simulink model "cps_physics_v2"  (R2012b)
settings: Solver=FixedStepDiscrete  StartTime=0.0  StopTime=8.5  FixedStep=0.005  RelTol=1e-5
model workspace (MAT data in the model file):
  nozzle_radius = 0.06
  block_mass = 0.0075
  block_width = 0.15
  ini_G_block_hpos = -0.4
  ini_G_block_vpos = 0.11
  ini_nozzle_pos = 0.3
  block_height = 0.1
  board_vpos = -0.1
  ini_R_block_hpos = -0.4
  ini_R_block_vpos = 0.01
  ini_B_block_vpos = 0.21
  ini_B_block_hpos = -0.4
libraries: fl_lib x52, nesl_utility x19, cps_physics_lib x4, cps_lib_v2 x3
settings Model: Creator=pmosterm  LastModifiedBy=pmosterm
settings SolverCC: MaxConsecutiveZCs=100  EnableConcurrentExecution=on  ConcurrentTasks=on  ZeroCrossAlgorithm=Adaptive
settings DataIOCC: SignalLoggingSaveFormat=ModelDataLogs  SaveOutput=off  DSMLogging=off  SaveTime=off
settings OptimizationCC: InlineParams=on
settings DebuggingCC: ReadBeforeWriteMsg=DisableAll  WriteAfterWriteMsg=DisableAll  WriteAfterReadMsg=DisableAll  AlgebraicLoopMsg=error  UnderspecifiedInitializationDetection=Simplified  FcnCallInpInsideContextMsg=EnableAllAsWarning  ModelReferenceExtraNoncontSigs=warning
settings GRTTargetCC: CombineOutputUpdateFcns=off  GRTInterface=on

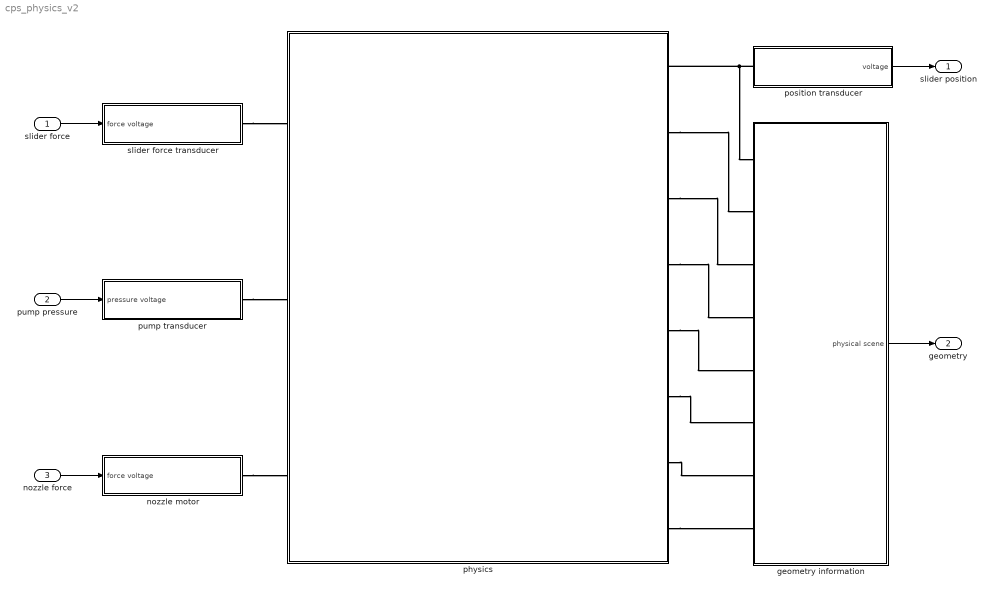
== system cps_physics_v2 ==
  slider force : Inport  SampleTime=[0 1]
  pump pressure : Inport  Port=2
  nozzle force : Inport  Port=3
  geometry information : Subsystem
  nozzle motor : Subsystem
  physics : Subsystem
      settings: OpenFcn=open_system(gcb,'force');
      mask Display: image(imread('images\geo_ton_428x599.jpg'));
  position transducer : Subsystem
  pump transducer : Subsystem
  slider force transducer : Subsystem
  slider position : Outport
  geometry : Outport  Port=2  OutDataTypeStr=Bus: slBusGeometry  BusOutputAsStruct=on
  wires:
  slider force/1 -> slider force transducer/1(force voltage)
  nozzle force/1 -> nozzle motor/1(force voltage)
  pump pressure/1 -> pump transducer/1(pressure voltage)
  geometry information/1(physical scene) -> geometry/1
  position transducer/1(voltage) -> slider position/1
  connections:
  position transducer/LConn1 -- physics/RConn1 -- geometry information/LConn1
  nozzle motor/RConn1 -- physics/LConn3
  physics/RConn4 -- geometry information/LConn4
  physics/RConn3 -- geometry information/LConn3
  slider force transducer/RConn1 -- physics/LConn1
  pump transducer/RConn1 -- physics/LConn2
  physics/RConn2 -- geometry information/LConn2
  physics/RConn5 -- geometry information/LConn5
  physics/RConn6 -- geometry information/LConn6
  physics/RConn7 -- geometry information/LConn7
  physics/RConn8 -- geometry information/LConn8

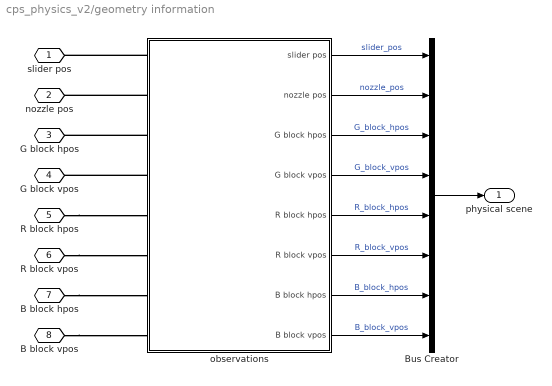
== system cps_physics_v2/geometry information ==
  Bus Creator : BusCreator  Inputs='slider_pos','nozzle_pos','G_block_hpos','G_block_vpos','R_block_hpos','R_block_vpos','B_block_hpos','B_block_vpos'
  observations : Subsystem
  slider pos : PMIOPort  Port=1  Side=Left
  nozzle pos : PMIOPort  Port=2  Side=Left
  G block hpos : PMIOPort  Port=3  Side=Left
  G block vpos : PMIOPort  Port=4  Side=Left
  R block hpos : PMIOPort  Port=5  Side=Left
  R block vpos : PMIOPort  Port=6  Side=Left
  B block hpos : PMIOPort  Port=7  Side=Left
  B block vpos : PMIOPort  Port=8  Side=Left
  physical scene : Outport  OutDataTypeStr=Bus: slBusGeometry
  wires:
  Bus Creator/1 -> physical scene/1
  observations/2(nozzle pos) -> Bus Creator/2  "nozzle_pos"
  observations/3(G block hpos) -> Bus Creator/3  "G_block_hpos"
  observations/4(G block vpos) -> Bus Creator/4  "G_block_vpos"
  observations/1(slider pos) -> Bus Creator/1  "slider_pos"
  observations/5(R block hpos) -> Bus Creator/5  "R_block_hpos"
  observations/6(R block vpos) -> Bus Creator/6  "R_block_vpos"
  observations/7(B block hpos) -> Bus Creator/7  "B_block_hpos"
  observations/8(B block vpos) -> Bus Creator/8  "B_block_vpos"
  connections:
  observations/LConn4 -- G block vpos/RConn1
  observations/LConn3 -- G block hpos/RConn1
  observations/LConn1 -- slider pos/RConn1
  observations/LConn2 -- nozzle pos/RConn1
  R block vpos/RConn1 -- observations/LConn6
  R block hpos/RConn1 -- observations/LConn5
  B block hpos/RConn1 -- observations/LConn7
  B block vpos/RConn1 -- observations/LConn8

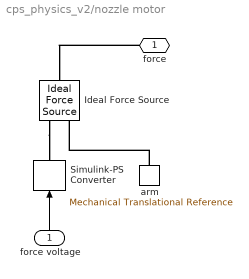
== system cps_physics_v2/nozzle motor ==
  force voltage : Inport
  Ideal Force Source : fl_lib/Mechanical/Mechanical Sources/Ideal Force Source  v_Log=off  f_Log=off  LocalVarNames=|v|f  LocalVarDescs=|v|f  LocalVarLogging=[0 0]
  Simulink-PS Converter : nesl_utility/Simulink-PS Converter  PhysicalDomain=network_engine_domain  LeftPortType=input  RightPortType=output  SubClassName=ps_input  PseudoPeriodic=off  Frequencies=[]  NoiseDistribution=none  NoiseParameters=[]  Unit=1  AffineConversion=off  InputFilterTimeConstant=.001  UdotUserProvided=0  SimscapeFilterOrder=1  InputFiltering=off
  arm : fl_lib/Mechanical/Translational Elements/Mechanical Translational Reference  f_Log=off  LocalVarNames=|f  LocalVarDescs=|f  LocalVarLogging=0
  force : PMIOPort  Port=1  Side=Right
  wires:
  force voltage/1 -> Simulink-PS Converter/1
  connections:
  Ideal Force Source/RConn1 -- Simulink-PS Converter/RConn1
  force/RConn1 -- Ideal Force Source/LConn1
  arm/LConn1 -- Ideal Force Source/RConn2

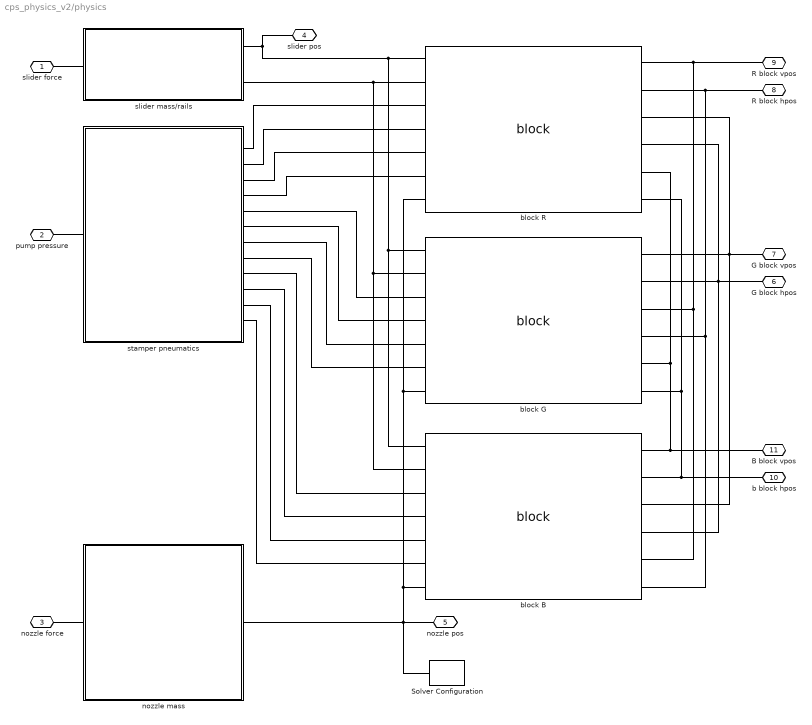
== system cps_physics_v2/physics ==
  Solver Configuration : nesl_utility/Solver Configuration  PhysicalDomain=network_engine_domain  LeftPortType=input  RightPortType=generic  SubClassName=solver  Accelerate=off  Profile=off  UseLocalSampling=off  FrequencyDomain=off  Tones=[]  Harmonics=[]  UseCCode=off  SimulateNoise=off  EnableSwitchedLinearOptims=on  DoDC=off  ResidualTolerance=1e-9  UseLocalSolver=on  LocalSolverChoice=NE_BACKWARD_EULER_ADVANCER  LocalSolverSampleTime=.005  DoFixedCost=on  MaxNonlinIter=3  MaxModeIter=2  LinearAlgebra=Sparse  DelaysMemoryBudget=1024
  block B : cps_lib_v2/block  ini_block_vpos=ini_B_block_vpos  ini_block_hpos=ini_B_block_hpos
  block G : cps_lib_v2/block  ini_block_vpos=ini_G_block_vpos  ini_block_hpos=ini_G_block_hpos
  block R : cps_lib_v2/block  ini_block_vpos=ini_R_block_vpos  ini_block_hpos=ini_R_block_hpos
  nozzle mass : Subsystem
      settings: OpenFcn=open_system(gcb,'force');
      mask Display: image(imread('images\geo_ton_slider_nozzle_202x195.jpg'));
  slider mass/rails : Subsystem
      settings: OpenFcn=open_system(gcb,'force');
      mask Display: image(imread('images\geo_ton_slider_rails_202x88.jpg'));
  stamper pneumatics : Subsystem
      settings: OpenFcn=open_system(gcb,'force');
      mask Display: image(imread('images\geo_ton_pneumatics_202x264.jpg'));
  slider force : PMIOPort  Port=1  Side=Left
  pump pressure : PMIOPort  Port=2  Side=Left
  nozzle force : PMIOPort  Port=3  Side=Left
  slider pos : PMIOPort  Port=4  Side=Right
  nozzle pos : PMIOPort  Port=5  Side=Right
  G block hpos : PMIOPort  Port=6  Side=Right
  G block vpos : PMIOPort  Port=7  Side=Right
  R block hpos : PMIOPort  Port=8  Side=Right
  R block vpos : PMIOPort  Port=9  Side=Right
  b block hpos : PMIOPort  Port=10  Side=Right
  B block vpos : PMIOPort  Port=11  Side=Right
  connections:
  slider mass/rails/RConn1 -- block R/LConn1 -- block B/LConn1 -- block G/LConn1 -- slider pos/RConn1
  slider force/RConn1 -- slider mass/rails/LConn1
  pump pressure/RConn1 -- stamper pneumatics/LConn1
  nozzle force/RConn1 -- nozzle mass/LConn1
  G block hpos/RConn1 -- block B/RConn4 -- block G/RConn2 -- block R/RConn4
  block R/LConn2 -- slider mass/rails/RConn2 -- block B/LConn2 -- block G/LConn2
  R block vpos/RConn1 -- block R/RConn1 -- block B/RConn5 -- block G/RConn3
  R block hpos/RConn1 -- block R/RConn2 -- block B/RConn6 -- block G/RConn4
  G block vpos/RConn1 -- block B/RConn3 -- block G/RConn1 -- block R/RConn3
  nozzle pos/RConn1 -- Solver Configuration/RConn1 -- nozzle mass/RConn1 -- block G/LConn7 -- block R/LConn7 -- block B/LConn7
  block G/LConn3 -- stamper pneumatics/RConn5
  block G/LConn4 -- stamper pneumatics/RConn6
  block G/LConn5 -- stamper pneumatics/RConn7
  block G/LConn6 -- stamper pneumatics/RConn8
  block R/LConn5 -- stamper pneumatics/RConn3
  block R/LConn3 -- stamper pneumatics/RConn1
  block R/LConn4 -- stamper pneumatics/RConn2
  block R/LConn6 -- stamper pneumatics/RConn4
  block B/LConn3 -- stamper pneumatics/RConn9
  block B/LConn4 -- stamper pneumatics/RConn10
  block B/LConn5 -- stamper pneumatics/RConn11
  block B/LConn6 -- stamper pneumatics/RConn12
  B block vpos/RConn1 -- block G/RConn5 -- block R/RConn5 -- block B/RConn1
  b block hpos/RConn1 -- block G/RConn6 -- block R/RConn6 -- block B/RConn2

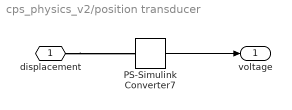
== system cps_physics_v2/position transducer ==
  PS-Simulink Converter7 : nesl_utility/PS-Simulink Converter  PhysicalDomain=network_engine_domain  LeftPortType=input  RightPortType=output  SubClassName=ps_output  PseudoPeriodic=off  Frequencies=[]  Unit=1  AffineConversion=off
  displacement : PMIOPort  Port=1  Side=Left
  voltage : Outport
  wires:
  PS-Simulink Converter7/1 -> voltage/1
  connections:
  displacement/RConn1 -- PS-Simulink Converter7/LConn1

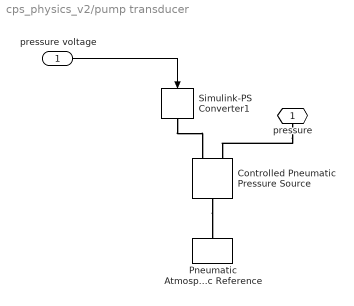
== system cps_physics_v2/pump transducer ==
  pressure voltage : Inport
  Controlled Pneumatic Pressure Source : fl_lib/Pneumatic/Pneumatic Sources/Controlled Pneumatic Pressure Source  pressure_difference_Log=off  gas_flow_Log=off  temperature_difference_Log=off  heat_flow_Log=off  LocalVarNames=|pressure_difference|gas_flow|temperature_difference|heat_flow  LocalVarDescs=|pressure_difference|gas_flow|temperature_difference|heat_flow  LocalVarLogging=[0 0 0 0]
  Pneumatic Atmospheric Reference : fl_lib/Pneumatic/Pneumatic Elements/Pneumatic Atmospheric Reference  gas_flow_Log=off  heat_flow_Log=off  LocalVarNames=|gas_flow|heat_flow  LocalVarDescs=|gas_flow|heat_flow  LocalVarLogging=[0 0]
  Simulink-PS Converter1 : nesl_utility/Simulink-PS Converter  PhysicalDomain=network_engine_domain  LeftPortType=input  RightPortType=output  SubClassName=ps_input  PseudoPeriodic=off  Frequencies=[]  NoiseDistribution=none  NoiseParameters=[]  Unit=1  AffineConversion=off  InputFilterTimeConstant=.001  UdotUserProvided=0  SimscapeFilterOrder=1  InputFiltering=off
  pressure : PMIOPort  Port=1  Side=Right
  wires:
  pressure voltage/1 -> Simulink-PS Converter1/1
  connections:
  pressure/RConn1 -- Controlled Pneumatic Pressure Source/RConn1
  Controlled Pneumatic Pressure Source/LConn1 -- Pneumatic Atmospheric Reference/LConn1
  Simulink-PS Converter1/RConn1 -- Controlled Pneumatic Pressure Source/RConn2

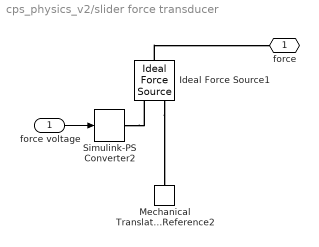
== system cps_physics_v2/slider force transducer ==
  force voltage : Inport
  Ideal Force Source1 : fl_lib/Mechanical/Mechanical Sources/Ideal Force Source  v_Log=off  f_Log=off  LocalVarNames=|v|f  LocalVarDescs=|v|f  LocalVarLogging=[0 0]
  Mechanical Translational Reference2 : fl_lib/Mechanical/Translational Elements/Mechanical Translational Reference  f_Log=off  LocalVarNames=|f  LocalVarDescs=|f  LocalVarLogging=0
  Simulink-PS Converter2 : nesl_utility/Simulink-PS Converter  PhysicalDomain=network_engine_domain  LeftPortType=input  RightPortType=output  SubClassName=ps_input  PseudoPeriodic=off  Frequencies=[]  NoiseDistribution=none  NoiseParameters=[]  Unit=1  AffineConversion=off  InputFilterTimeConstant=.001  UdotUserProvided=0  SimscapeFilterOrder=1  InputFiltering=off
  force : PMIOPort  Port=1  Side=Right
  wires:
  force voltage/1 -> Simulink-PS Converter2/1
  connections:
  Ideal Force Source1/RConn2 -- Mechanical Translational Reference2/LConn1
  Simulink-PS Converter2/RConn1 -- Ideal Force Source1/RConn1
  Ideal Force Source1/LConn1 -- force/RConn1

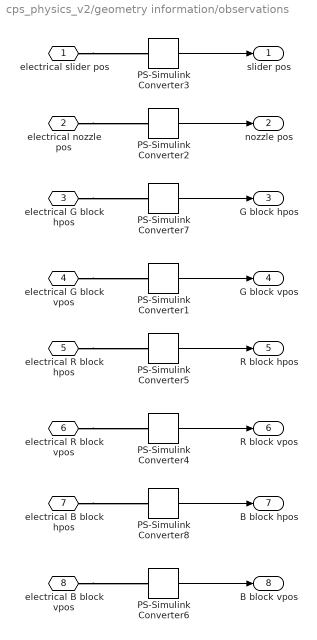
== system cps_physics_v2/geometry information/observations ==
  PS-Simulink Converter{1..8} (8 alike) : nesl_utility/PS-Simulink Converter  PhysicalDomain=network_engine_domain  LeftPortType=input  RightPortType=output  SubClassName=ps_output  PseudoPeriodic=off  Frequencies=[]  Unit=1  AffineConversion=off
  electrical slider pos : PMIOPort  Port=1  Side=Left
  electrical nozzle pos : PMIOPort  Port=2  Side=Left
  electrical G block hpos : PMIOPort  Port=3  Side=Left
  electrical G block vpos : PMIOPort  Port=4  Side=Left
  electrical R block hpos : PMIOPort  Port=5  Side=Left
  electrical R block vpos : PMIOPort  Port=6  Side=Left
  electrical B block hpos : PMIOPort  Port=7  Side=Left
  electrical B block vpos : PMIOPort  Port=8  Side=Left
  slider pos : Outport
  nozzle pos : Outport  Port=2
  G block hpos : Outport  Port=3
  G block vpos : Outport  Port=4
  R block hpos : Outport  Port=5
  R block vpos : Outport  Port=6
  B block hpos : Outport  Port=7
  B block vpos : Outport  Port=8
  wires:
  PS-Simulink Converter3/1 -> slider pos/1
  PS-Simulink Converter2/1 -> nozzle pos/1
  PS-Simulink Converter1/1 -> G block vpos/1
  PS-Simulink Converter7/1 -> G block hpos/1
  PS-Simulink Converter4/1 -> R block vpos/1
  PS-Simulink Converter5/1 -> R block hpos/1
  PS-Simulink Converter6/1 -> B block vpos/1
  PS-Simulink Converter8/1 -> B block hpos/1
  connections:
  electrical slider pos/RConn1 -- PS-Simulink Converter3/LConn1
  electrical nozzle pos/RConn1 -- PS-Simulink Converter2/LConn1
  electrical G block vpos/RConn1 -- PS-Simulink Converter1/LConn1
  electrical G block hpos/RConn1 -- PS-Simulink Converter7/LConn1
  electrical R block hpos/RConn1 -- PS-Simulink Converter5/LConn1
  electrical R block vpos/RConn1 -- PS-Simulink Converter4/LConn1
  electrical B block vpos/RConn1 -- PS-Simulink Converter6/LConn1
  electrical B block hpos/RConn1 -- PS-Simulink Converter8/LConn1

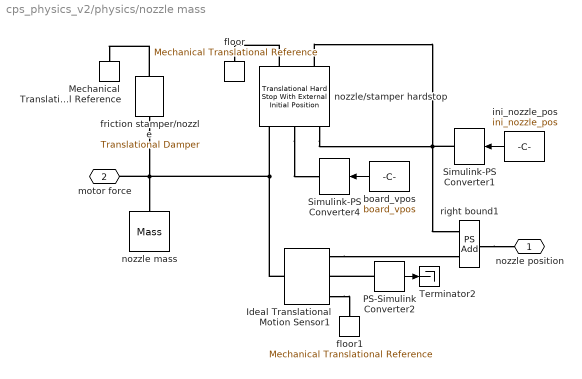
== system cps_physics_v2/physics/nozzle mass ==
  Ideal Translational Motion Sensor1 : fl_lib/Mechanical/Mechanical Sensors/Ideal Translational Motion Sensor  offset=0 m  v_Log=off  f_Log=off  x_Log=off  LocalVarNames=|v|f|x  LocalVarDescs=|v|f|x  LocalVarLogging=[0 0 0]
  Mechanical Translational Reference : fl_lib/Mechanical/Translational Elements/Mechanical Translational Reference  f_Log=off  LocalVarNames=|f  LocalVarDescs=|f  LocalVarLogging=0
  PS-Simulink Converter2 : nesl_utility/PS-Simulink Converter  PhysicalDomain=network_engine_domain  LeftPortType=input  RightPortType=output  SubClassName=ps_output  PseudoPeriodic=off  Frequencies=[]  Unit=1  AffineConversion=off
  Simulink-PS Converter1 : nesl_utility/Simulink-PS Converter  PhysicalDomain=network_engine_domain  LeftPortType=input  RightPortType=output  SubClassName=ps_input  PseudoPeriodic=off  Frequencies=[]  NoiseDistribution=none  NoiseParameters=[]  Unit=1  AffineConversion=off  InputFilterTimeConstant=.001  UdotUserProvided=[]  SimscapeFilterOrder=1  InputFiltering=off
  Simulink-PS Converter4 : nesl_utility/Simulink-PS Converter  PhysicalDomain=network_engine_domain  LeftPortType=input  RightPortType=output  SubClassName=ps_input  PseudoPeriodic=off  Frequencies=[]  NoiseDistribution=none  NoiseParameters=[]  Unit=1  AffineConversion=off  InputFilterTimeConstant=.001  UdotUserProvided=[]  SimscapeFilterOrder=1  InputFiltering=off
  Terminator2 : Terminator
  board_vpos : Constant  Value=board_vpos
  floor : fl_lib/Mechanical/Translational Elements/Mechanical Translational Reference  f_Log=off  LocalVarNames=|f  LocalVarDescs=|f  LocalVarLogging=0
  floor1 : fl_lib/Mechanical/Translational Elements/Mechanical Translational Reference  f_Log=off  LocalVarNames=|f  LocalVarDescs=|f  LocalVarLogging=0
  friction stamper/nozzle : fl_lib/Mechanical/Translational Elements/Translational Damper  D=100 N/(m/s)  f_Log=off  v_Log=off  LocalVarNames=|f|v  LocalVarDescs=|f|v  LocalVarLogging=[0 0]
  ini_nozzle_pos : Constant  Value=ini_nozzle_pos
  nozzle mass : fl_lib/Mechanical/Translational Elements/Mass  mass=0.5 kg  initial_velocity=0 m/s  f_Log=off  LocalVarNames=|f  LocalVarDescs=|f  LocalVarLogging=0
  nozzle/stamper hardstop : cps_physics_lib/Translational Hard Stop With External Initial Position  stiff_up=1e4 N/m  stiff_low=1e6 N/m  D_up=150 N/(m/s)  D_low=150 N/(m/s)  f_Log=off  v_Log=off  x_Log=off  LocalVarNames=|f|v|x  LocalVarDescs=|f|v|x  LocalVarLogging=[0 0 0]
  right bound1 : fl_lib/Physical Signals/Functions/PS Add  LocalVarLogging=[]
  nozzle position : PMIOPort  Port=1  Side=Right
  motor force : PMIOPort  Port=2  Side=Left
  wires:
  board_vpos/1 -> Simulink-PS Converter4/1
  PS-Simulink Converter2/1 -> Terminator2/1
  ini_nozzle_pos/1 -> Simulink-PS Converter1/1
  connections:
  nozzle/stamper hardstop/RConn1 -- floor/LConn1
  Ideal Translational Motion Sensor1/LConn1 -- nozzle/stamper hardstop/LConn1 -- nozzle mass/LConn1 -- motor force/RConn1 -- friction stamper/nozzle/LConn1
  right bound1/RConn1 -- nozzle position/RConn1
  friction stamper/nozzle/RConn1 -- Mechanical Translational Reference/LConn1
  nozzle/stamper hardstop/LConn2 -- Simulink-PS Converter4/RConn1
  Ideal Translational Motion Sensor1/RConn1 -- floor1/LConn1
  nozzle/stamper hardstop/RConn2 -- nozzle/stamper hardstop/LConn3 -- Simulink-PS Converter1/RConn1 -- right bound1/LConn2
  Ideal Translational Motion Sensor1/RConn3 -- right bound1/LConn1
  PS-Simulink Converter2/LConn1 -- Ideal Translational Motion Sensor1/RConn2

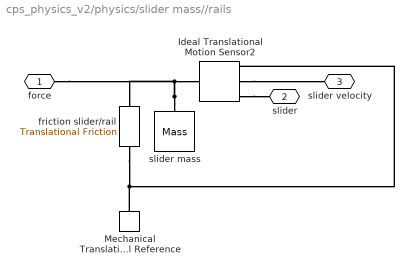
== system cps_physics_v2/physics/slider mass//rails ==
  Ideal Translational Motion Sensor2 : fl_lib/Mechanical/Mechanical Sensors/Ideal Translational Motion Sensor  offset=0 m  v_Log=off  f_Log=off  x_Log=off  LocalVarNames=|v|f|x  LocalVarDescs=|v|f|x  LocalVarLogging=[0 0 0]
  Mechanical Translational Reference : fl_lib/Mechanical/Translational Elements/Mechanical Translational Reference  f_Log=off  LocalVarNames=|f  LocalVarDescs=|f  LocalVarLogging=0
  friction slider/rail : fl_lib/Mechanical/Translational Elements/Translational Friction  brkwy_frc=2.5 N  Col_frc=2 N  visc_coef=10 N/(m/s)  trans_coef=1 s/m  vel_thr=1e-5 m/s  f_Log=off  v_Log=off  LocalVarNames=|f|v  LocalVarDescs=|f|v  LocalVarLogging=[0 0]
  slider mass : fl_lib/Mechanical/Translational Elements/Mass  mass=1 kg  initial_velocity=0 m/s  f_Log=off  LocalVarNames=|f  LocalVarDescs=|f  LocalVarLogging=0
  force : PMIOPort  Port=1  Side=Left
  slider : PMIOPort  Port=2  Side=Right
  slider velocity : PMIOPort  Port=3  Side=Right
  connections:
  Ideal Translational Motion Sensor2/RConn3 -- slider/RConn1
  Mechanical Translational Reference/LConn1 -- Ideal Translational Motion Sensor2/RConn1 -- friction slider/rail/RConn1
  slider mass/LConn1 -- Ideal Translational Motion Sensor2/LConn1 -- force/RConn1 -- friction slider/rail/LConn1
  Ideal Translational Motion Sensor2/RConn2 -- slider velocity/RConn1

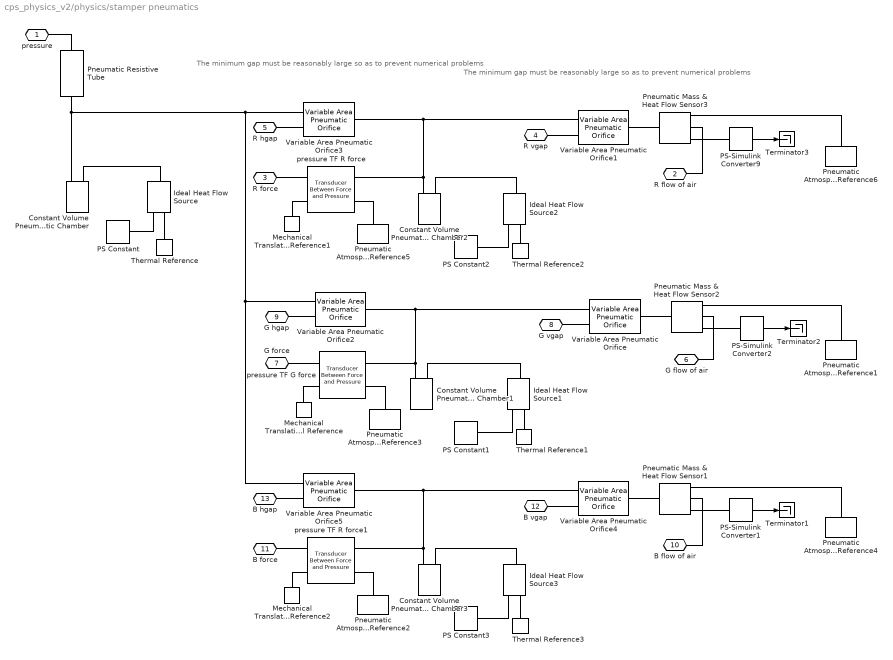
== system cps_physics_v2/physics/stamper pneumatics ==
  note: The minimum gap must be
      | reasonably large
      | so as to prevent
      | numerical problems
  note: The minimum gap must be
      | reasonably large
      | so as to prevent
      | numerical problems
  Constant Volume Pneumatic Chamber : fl_lib/Pneumatic/Pneumatic Elements/Constant Volume Pneumatic Chamber  Volume=7e-6 m^3  p0=101325 Pa  T0=293.15 K  gas_flow_Log=off  heat_flow_Log=off  pressure_Log=off  temperature_Log=off  gas_temperature_Log=off  heat_exch_flow_Log=off  LocalVarNames=|gas_flow|heat_flow|pressure|temperature|heat_exch_flow|wall_temperature  LocalVarDescs=|gas_flow|heat_flow|pressure|temperature|heat_exch_flow|wall_temperature  LocalVarLogging=[0 0 0 0 0 0]
  Constant Volume Pneumatic Chamber1 : fl_lib/Pneumatic/Pneumatic Elements/Constant Volume Pneumatic Chamber  Volume=14e-4 m^3  p0=101325 Pa  T0=293.15 K  gas_flow_Log=off  heat_flow_Log=off  pressure_Log=off  temperature_Log=off  gas_temperature_Log=off  heat_exch_flow_Log=off  LocalVarNames=|gas_flow|heat_flow|pressure|temperature|heat_exch_flow|wall_temperature  LocalVarDescs=|gas_flow|heat_flow|pressure|temperature|heat_exch_flow|wall_temperature  LocalVarLogging=[0 0 0 0 0 0]
  Constant Volume Pneumatic Chamber2 : fl_lib/Pneumatic/Pneumatic Elements/Constant Volume Pneumatic Chamber  Volume=14e-4 m^3  p0=101325 Pa  T0=293.15 K  gas_flow_Log=off  heat_flow_Log=off  pressure_Log=off  temperature_Log=off  gas_temperature_Log=off  heat_exch_flow_Log=off  LocalVarNames=|gas_flow|heat_flow|pressure|temperature|heat_exch_flow|wall_temperature  LocalVarDescs=|gas_flow|heat_flow|pressure|temperature|heat_exch_flow|wall_temperature  LocalVarLogging=[0 0 0 0 0 0]
  Constant Volume Pneumatic Chamber3 : fl_lib/Pneumatic/Pneumatic Elements/Constant Volume Pneumatic Chamber  Volume=14e-4 m^3  p0=101325 Pa  T0=293.15 K  gas_flow_Log=off  heat_flow_Log=off  pressure_Log=off  temperature_Log=off  gas_temperature_Log=off  heat_exch_flow_Log=off  LocalVarNames=|gas_flow|heat_flow|pressure|temperature|heat_exch_flow|wall_temperature  LocalVarDescs=|gas_flow|heat_flow|pressure|temperature|heat_exch_flow|wall_temperature  LocalVarLogging=[0 0 0 0 0 0]
  Ideal Heat Flow Source{,1..3} (4 alike) : fl_lib/Thermal/Thermal Sources/Ideal Heat Flow Source  Q_Log=off  T_Log=off  LocalVarNames=|Q|T  LocalVarDescs=|Q|T  LocalVarLogging=[0 0]
  Mechanical Translational Reference : fl_lib/Mechanical/Translational Elements/Mechanical Translational Reference  f_Log=off  LocalVarNames=|f  LocalVarDescs=|f  LocalVarLogging=0
  Mechanical Translational Reference1 : fl_lib/Mechanical/Translational Elements/Mechanical Translational Reference  f_Log=off  LocalVarNames=|f  LocalVarDescs=|f  LocalVarLogging=0
  Mechanical Translational Reference2 : fl_lib/Mechanical/Translational Elements/Mechanical Translational Reference  f_Log=off  LocalVarNames=|f  LocalVarDescs=|f  LocalVarLogging=0
  PS Constant{,1..3} (4 alike) : fl_lib/Physical Signals/Sources/PS Constant  constant=0  LocalVarLogging=[]
  PS-Simulink Converter1 : nesl_utility/PS-Simulink Converter  PhysicalDomain=network_engine_domain  LeftPortType=input  RightPortType=output  SubClassName=ps_output  PseudoPeriodic=off  Frequencies=[]  Unit=1  AffineConversion=off
  PS-Simulink Converter2 : nesl_utility/PS-Simulink Converter  PhysicalDomain=network_engine_domain  LeftPortType=input  RightPortType=output  SubClassName=ps_output  PseudoPeriodic=off  Frequencies=[]  Unit=1  AffineConversion=off
  PS-Simulink Converter9 : nesl_utility/PS-Simulink Converter  PhysicalDomain=network_engine_domain  LeftPortType=input  RightPortType=output  SubClassName=ps_output  PseudoPeriodic=off  Frequencies=[]  Unit=1  AffineConversion=off
  Pneumatic Atmospheric Reference{1..6} (6 alike) : fl_lib/Pneumatic/Pneumatic Elements/Pneumatic Atmospheric Reference  gas_flow_Log=off  heat_flow_Log=off  LocalVarNames=|gas_flow|heat_flow  LocalVarDescs=|gas_flow|heat_flow  LocalVarLogging=[0 0]
  Pneumatic Mass & Heat Flow Sensor1 : fl_lib/Pneumatic/Pneumatic Sensors/Pneumatic Mass & Heat Flow Sensor  pressure_difference_Log=off  gas_flow_Log=off  temperature_difference_Log=off  heat_flow_Log=off  LocalVarNames=|pressure_difference|gas_flow|temperature_difference|heat_flow  LocalVarDescs=|pressure_difference|gas_flow|temperature_difference|heat_flow  LocalVarLogging=[0 0 0 0]
  Pneumatic Mass & Heat Flow Sensor2 : fl_lib/Pneumatic/Pneumatic Sensors/Pneumatic Mass & Heat Flow Sensor  pressure_difference_Log=off  gas_flow_Log=off  temperature_difference_Log=off  heat_flow_Log=off  LocalVarNames=|pressure_difference|gas_flow|temperature_difference|heat_flow  LocalVarDescs=|pressure_difference|gas_flow|temperature_difference|heat_flow  LocalVarLogging=[0 0 0 0]
  Pneumatic Mass & Heat Flow Sensor3 : fl_lib/Pneumatic/Pneumatic Sensors/Pneumatic Mass & Heat Flow Sensor  pressure_difference_Log=off  gas_flow_Log=off  temperature_difference_Log=off  heat_flow_Log=off  LocalVarNames=|pressure_difference|gas_flow|temperature_difference|heat_flow  LocalVarDescs=|pressure_difference|gas_flow|temperature_difference|heat_flow  LocalVarLogging=[0 0 0 0]
  Pneumatic Resistive Tube : fl_lib/Pneumatic/Pneumatic Elements/Pneumatic Resistive Tube  Diameter=1e-2 m  Length=4e-2 m  EquivalentLength=0 m  Roughness=1.5e-5 m  Re_lam=2300  Re_turb=4000  G_Log=off  Q1_Log=off  Q2_Log=off  p1_Log=off  p2_Log=off  T1_Log=off  T2_Log=off  LocalVarNames=|G|Q1|Q2|p1|p2|T1|T2  LocalVarDescs=|G|Q1|Q2|p1|p2|T1|T2  LocalVarLogging=[0 0 0 0 0 0 0]
  Terminator1 : Terminator
  Terminator2 : Terminator
  Terminator3 : Terminator
  Thermal Reference{,1..3} (4 alike) : fl_lib/Thermal/Thermal Elements/Thermal Reference  Q_Log=off  LocalVarNames=|Q  LocalVarDescs=|Q  LocalVarLogging=0
  Variable Area Pneumatic Orifice : fl_lib/Pneumatic/Pneumatic Elements/Variable Area Pneumatic Orifice  Cd=0.82  Area0=4e-3 m^2  G_Log=off  Q1_Log=off  Q2_Log=off  p1_Log=off  p2_Log=off  T1_Log=off  T2_Log=off  LocalVarNames=|G|Q1|Q2|p1|p2|T1|T2  LocalVarDescs=|G|Q1|Q2|p1|p2|T1|T2  LocalVarLogging=[0 0 0 0 0 0 0]
  Variable Area Pneumatic Orifice1 : fl_lib/Pneumatic/Pneumatic Elements/Variable Area Pneumatic Orifice  Cd=0.82  Area0=4e-3 m^2  G_Log=off  Q1_Log=off  Q2_Log=off  p1_Log=off  p2_Log=off  T1_Log=off  T2_Log=off  LocalVarNames=|G|Q1|Q2|p1|p2|T1|T2  LocalVarDescs=|G|Q1|Q2|p1|p2|T1|T2  LocalVarLogging=[0 0 0 0 0 0 0]
  Variable Area Pneumatic Orifice2 : fl_lib/Pneumatic/Pneumatic Elements/Variable Area Pneumatic Orifice  Cd=0.82  Area0=1e-4 m^2  G_Log=off  Q1_Log=off  Q2_Log=off  p1_Log=off  p2_Log=off  T1_Log=off  T2_Log=off  LocalVarNames=|G|Q1|Q2|p1|p2|T1|T2  LocalVarDescs=|G|Q1|Q2|p1|p2|T1|T2  LocalVarLogging=[0 0 0 0 0 0 0]
  Variable Area Pneumatic Orifice3 : fl_lib/Pneumatic/Pneumatic Elements/Variable Area Pneumatic Orifice  Cd=0.82  Area0=1e-4 m^2  G_Log=off  Q1_Log=off  Q2_Log=off  p1_Log=off  p2_Log=off  T1_Log=off  T2_Log=off  LocalVarNames=|G|Q1|Q2|p1|p2|T1|T2  LocalVarDescs=|G|Q1|Q2|p1|p2|T1|T2  LocalVarLogging=[0 0 0 0 0 0 0]
  Variable Area Pneumatic Orifice4 : fl_lib/Pneumatic/Pneumatic Elements/Variable Area Pneumatic Orifice  Cd=0.82  Area0=4e-3 m^2  G_Log=off  Q1_Log=off  Q2_Log=off  p1_Log=off  p2_Log=off  T1_Log=off  T2_Log=off  LocalVarNames=|G|Q1|Q2|p1|p2|T1|T2  LocalVarDescs=|G|Q1|Q2|p1|p2|T1|T2  LocalVarLogging=[0 0 0 0 0 0 0]
  Variable Area Pneumatic Orifice5 : fl_lib/Pneumatic/Pneumatic Elements/Variable Area Pneumatic Orifice  Cd=0.82  Area0=1e-4 m^2  G_Log=off  Q1_Log=off  Q2_Log=off  p1_Log=off  p2_Log=off  T1_Log=off  T2_Log=off  LocalVarNames=|G|Q1|Q2|p1|p2|T1|T2  LocalVarDescs=|G|Q1|Q2|p1|p2|T1|T2  LocalVarLogging=[0 0 0 0 0 0 0]
  pressure TF G force : cps_physics_lib/Transducer Between Force and Pressure  area=-pi*nozzle_radius*nozzle_radius  p1_Log=off  f2_Log=off  G1_Log=off  v2_Log=off  T1_Log=off  Q1_Log=off  heat_flow_Log=off  LocalVarNames=|p1|f2|G1|v2|T1|Q1|heat_flow  LocalVarDescs=|p1|f2|G1|v2|T1|Q1|heat_flow  LocalVarLogging=[0 0 0 0 0 0 0]
  pressure TF R force : cps_physics_lib/Transducer Between Force and Pressure  area=-pi*nozzle_radius*nozzle_radius  p1_Log=off  f2_Log=off  G1_Log=off  v2_Log=off  T1_Log=off  Q1_Log=off  heat_flow_Log=off  LocalVarNames=|p1|f2|G1|v2|T1|Q1|heat_flow  LocalVarDescs=|p1|f2|G1|v2|T1|Q1|heat_flow  LocalVarLogging=[0 0 0 0 0 0 0]
  pressure TF R force1 : cps_physics_lib/Transducer Between Force and Pressure  area=-pi*nozzle_radius*nozzle_radius  p1_Log=off  f2_Log=off  G1_Log=off  v2_Log=off  T1_Log=off  Q1_Log=off  heat_flow_Log=off  LocalVarNames=|p1|f2|G1|v2|T1|Q1|heat_flow  LocalVarDescs=|p1|f2|G1|v2|T1|Q1|heat_flow  LocalVarLogging=[0 0 0 0 0 0 0]
  pressure : PMIOPort  Port=1  Side=Left
  R flow of air : PMIOPort  Port=2  Side=Right
  R force : PMIOPort  Port=3  Side=Right
  R vgap : PMIOPort  Port=4  Side=Right
  R hgap : PMIOPort  Port=5  Side=Right
  G flow of air : PMIOPort  Port=6  Side=Right
  G force : PMIOPort  Port=7  Side=Right
  G vgap : PMIOPort  Port=8  Side=Right
  G hgap : PMIOPort  Port=9  Side=Right
  B flow of air : PMIOPort  Port=10  Side=Right
  B force : PMIOPort  Port=11  Side=Right
  B vgap : PMIOPort  Port=12  Side=Right
  B hgap : PMIOPort  Port=13  Side=Right
  wires:
  PS-Simulink Converter2/1 -> Terminator2/1
  PS-Simulink Converter9/1 -> Terminator3/1
  PS-Simulink Converter1/1 -> Terminator1/1
  connections:
  pressure TF G force/LConn2 -- Pneumatic Atmospheric Reference3/LConn1
  Constant Volume Pneumatic Chamber/LConn1 -- Variable Area Pneumatic Orifice3/LConn1 -- Variable Area Pneumatic Orifice5/LConn1 -- Variable Area Pneumatic Orifice2/LConn1 -- Pneumatic Resistive Tube/RConn1
  pressure TF G force/RConn2 -- Mechanical Translational Reference/LConn1
  G vgap/RConn1 -- Variable Area Pneumatic Orifice/LConn2
  Variable Area Pneumatic Orifice/RConn1 -- Pneumatic Mass & Heat Flow Sensor2/LConn1
  Pneumatic Mass & Heat Flow Sensor2/RConn1 -- Pneumatic Atmospheric Reference1/LConn1
  Pneumatic Mass & Heat Flow Sensor2/RConn2 -- G flow of air/RConn1
  PS-Simulink Converter2/LConn1 -- Pneumatic Mass & Heat Flow Sensor2/RConn3
  Constant Volume Pneumatic Chamber/LConn2 -- Ideal Heat Flow Source/LConn1
  Thermal Reference/LConn1 -- Ideal Heat Flow Source/RConn2
  PS Constant/RConn1 -- Ideal Heat Flow Source/RConn1
  pressure/RConn1 -- Pneumatic Resistive Tube/LConn1
  pressure TF G force/RConn1 -- G force/RConn1
  R vgap/RConn1 -- Variable Area Pneumatic Orifice1/LConn2
  Pneumatic Mass & Heat Flow Sensor3/LConn1 -- Variable Area Pneumatic Orifice1/RConn1
  pressure TF R force/RConn2 -- Mechanical Translational Reference1/LConn1
  pressure TF R force/LConn2 -- Pneumatic Atmospheric Reference5/LConn1
  pressure TF R force/RConn1 -- R force/RConn1
  R flow of air/RConn1 -- Pneumatic Mass & Heat Flow Sensor3/RConn2
  Pneumatic Mass & Heat Flow Sensor3/RConn3 -- PS-Simulink Converter9/LConn1
  Pneumatic Atmospheric Reference6/LConn1 -- Pneumatic Mass & Heat Flow Sensor3/RConn1
  Thermal Reference1/LConn1 -- Ideal Heat Flow Source1/RConn2
  Constant Volume Pneumatic Chamber1/LConn2 -- Ideal Heat Flow Source1/LConn1
  PS Constant1/RConn1 -- Ideal Heat Flow Source1/RConn1
  G hgap/RConn1 -- Variable Area Pneumatic Orifice2/LConn2
  Constant Volume Pneumatic Chamber1/LConn1 -- pressure TF G force/LConn1 -- Variable Area Pneumatic Orifice/LConn1 -- Variable Area Pneumatic Orifice2/RConn1
  R hgap/RConn1 -- Variable Area Pneumatic Orifice3/LConn2
  Thermal Reference2/LConn1 -- Ideal Heat Flow Source2/RConn2
  Ideal Heat Flow Source2/RConn1 -- PS Constant2/RConn1
  Constant Volume Pneumatic Chamber2/LConn2 -- Ideal Heat Flow Source2/LConn1
  Constant Volume Pneumatic Chamber2/LConn1 -- pressure TF R force/LConn1 -- Variable Area Pneumatic Orifice1/LConn1 -- Variable Area Pneumatic Orifice3/RConn1
  Constant Volume Pneumatic Chamber3/LConn1 -- Variable Area Pneumatic Orifice5/RConn1 -- Variable Area Pneumatic Orifice4/LConn1 -- pressure TF R force1/LConn1
  Constant Volume Pneumatic Chamber3/LConn2 -- Ideal Heat Flow Source3/LConn1
  Ideal Heat Flow Source3/RConn1 -- PS Constant3/RConn1
  Thermal Reference3/LConn1 -- Ideal Heat Flow Source3/RConn2
  B hgap/RConn1 -- Variable Area Pneumatic Orifice5/LConn2
  Pneumatic Atmospheric Reference4/LConn1 -- Pneumatic Mass & Heat Flow Sensor1/RConn1
  Pneumatic Mass & Heat Flow Sensor1/RConn3 -- PS-Simulink Converter1/LConn1
  B flow of air/RConn1 -- Pneumatic Mass & Heat Flow Sensor1/RConn2
  pressure TF R force1/RConn1 -- B force/RConn1
  pressure TF R force1/LConn2 -- Pneumatic Atmospheric Reference2/LConn1
  pressure TF R force1/RConn2 -- Mechanical Translational Reference2/LConn1
  Pneumatic Mass & Heat Flow Sensor1/LConn1 -- Variable Area Pneumatic Orifice4/RConn1
  B vgap/RConn1 -- Variable Area Pneumatic Orifice4/LConn2
